simulink model "GFLIB_ControllerPIpAW_BAM_F32"  (Simulink 8.3)
settings: Solver=ode45  StartTime=0.0  StopTime=10.0  RelTol=1e-3
undefined symbols (not defined in the file): f32IntegGain, f32PropGain, s16IntegGainShift, s16PropGainShift
settings Model: Creator=B17364  LastModifiedBy=B17364
settings DataIOCC: SignalLoggingSaveFormat=Dataset
settings DebuggingCC: UnderspecifiedInitializationDetection=Simplified  StateNameClashWarn=none
settings GRTTargetCC: CombineOutputUpdateFcns=on  GRTInterface=off

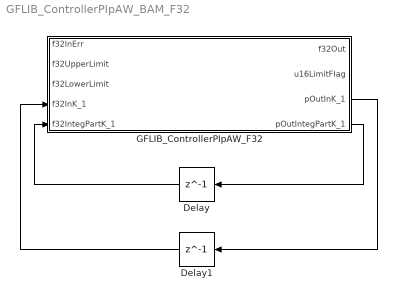
== system GFLIB_ControllerPIpAW_BAM_F32 ==
  Delay : Delay  DelayLength=1  InitialCondition=0
  Delay1 : Delay  DelayLength=1  InitialCondition=0
  GFLIB_ControllerPIpAW_F32 : Subsystem  mask(GFLIB_ControllerPIpAW_F32){f32PropGain=f32PropGain, s16PropGainShift=s16PropGainShift, f32IntegGain=f32IntegGain, s16IntegGainShift=s16IntegGainShift}
      mask help: Bit accurate model of parallel form PI controller with anti-windup. All parameters as well as input and output are 32-bit integers except for u16NShift parameter which is 16-bit unsigned integer.
      mask init:
      | pos = get_param(gcb, 'Position');width = pos(3) - pos(1); height = pos(4) - pos(2);tX=width/2;tY=height*0.9;
      mask Display: color('black');port_label('input',1,'f32InErr');port_label('input',2,'f32UpperLimit');port_label('input',3,'f32LowerLimit');port_label('input',4,'f32InK_1');port_label('input',5,'f32IntegPartK_1');port_label('output',1,'f32Out');port_label('output',2,'u16LimitFlag');port_label('output',3,'pOutInK_1');port_label('output',4,'pOutIntegPartK_1');color('black');disp('GFLIB_ControllerPIpAW_F32');color('blue');text(tX,tY, 'BAM', 'horizontalAlignment', 'center');
  wires:
  GFLIB_ControllerPIpAW_F32/4(pOutIntegPartK_1) -> Delay/1
  Delay/1 -> GFLIB_ControllerPIpAW_F32/5(f32IntegPartK_1)
  GFLIB_ControllerPIpAW_F32/3(pOutInK_1) -> Delay1/1
  Delay1/1 -> GFLIB_ControllerPIpAW_F32/4(f32InK_1)

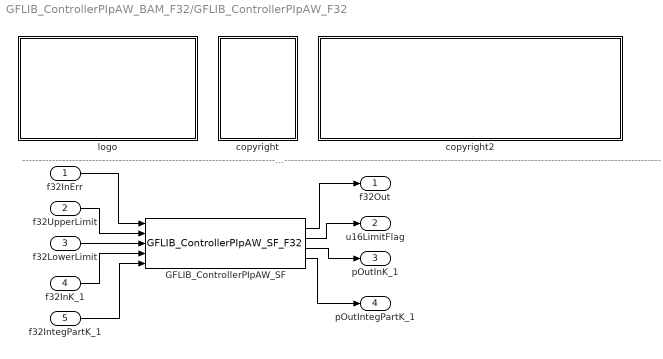
== system GFLIB_ControllerPIpAW_BAM_F32/GFLIB_ControllerPIpAW_F32 ==
  note: ---------------------------------------------------------------------------------------------------------------------------------------------------------------------------------------------------
  f32InErr : Inport
  f32UpperLimit : Inport  Port=2
  f32LowerLimit : Inport  Port=3
  f32InK_1 : Inport  Port=4
  f32IntegPartK_1 : Inport  Port=5
  GFLIB_ControllerPIpAW_SF : S-Function  FunctionName=GFLIB_ControllerPIpAW_SF_F32  Parameters=f32PropGain,s16PropGainShift,f32IntegGain,s16IntegGainShift  EnableBusSupport=off
  copyright : Subsystem
      mask Display: text(10,90,'FILE:');text(10,75,'DESRIPTION:');text(10,60,'COPYRIGHT:');text(10,45,'VERSION:');text(10,30,'DATE:')
  copyright2 : Subsystem
      mask Display: text(10,90,'GFLIB_ControllerPIpAW_BAM_F32.mdl');text(10,75,'Parallel form of a standard PI controller with implemented anti-windup.');text(10,60,'Freescale');text(10,45,'0.1');text(10,30,'12-Jun-2015');
  logo : Subsystem
      mask Display: image(imread('logo.jpg'))
  f32Out : Outport
  u16LimitFlag : Outport  Port=2
  pOutInK_1 : Outport  Port=3
  pOutIntegPartK_1 : Outport  Port=4
  wires:
  f32InErr/1 -> GFLIB_ControllerPIpAW_SF/1
  f32UpperLimit/1 -> GFLIB_ControllerPIpAW_SF/2
  f32LowerLimit/1 -> GFLIB_ControllerPIpAW_SF/3
  f32InK_1/1 -> GFLIB_ControllerPIpAW_SF/4
  f32IntegPartK_1/1 -> GFLIB_ControllerPIpAW_SF/5
  GFLIB_ControllerPIpAW_SF/1 -> f32Out/1
  GFLIB_ControllerPIpAW_SF/2 -> u16LimitFlag/1
  GFLIB_ControllerPIpAW_SF/3 -> pOutInK_1/1
  GFLIB_ControllerPIpAW_SF/4 -> pOutIntegPartK_1/1

== system GFLIB_ControllerPIpAW_BAM_F32/GFLIB_ControllerPIpAW_F32/copyright ==

== system GFLIB_ControllerPIpAW_BAM_F32/GFLIB_ControllerPIpAW_F32/copyright2 ==

== system GFLIB_ControllerPIpAW_BAM_F32/GFLIB_ControllerPIpAW_F32/logo ==
